simulink model "simulink_basic_blocks"  (R2022b)
settings: Solver=VariableStepAuto  StartTime=0.0  StopTime=10.0  RelTol=1e-3
settings Model: Creator=Soliman Rabie  LastModifiedBy=Soliman Rabie

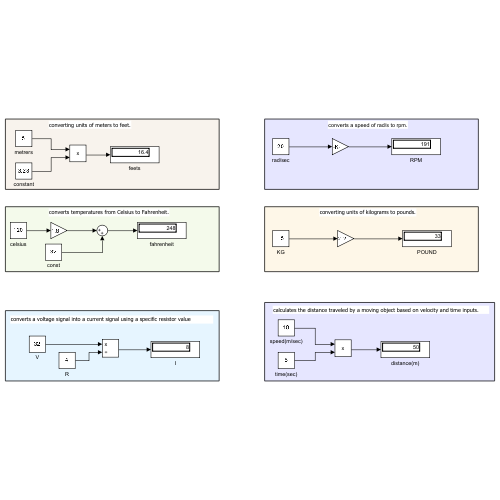
[thumbnail: Simulink's stored preview of the top-level diagram]
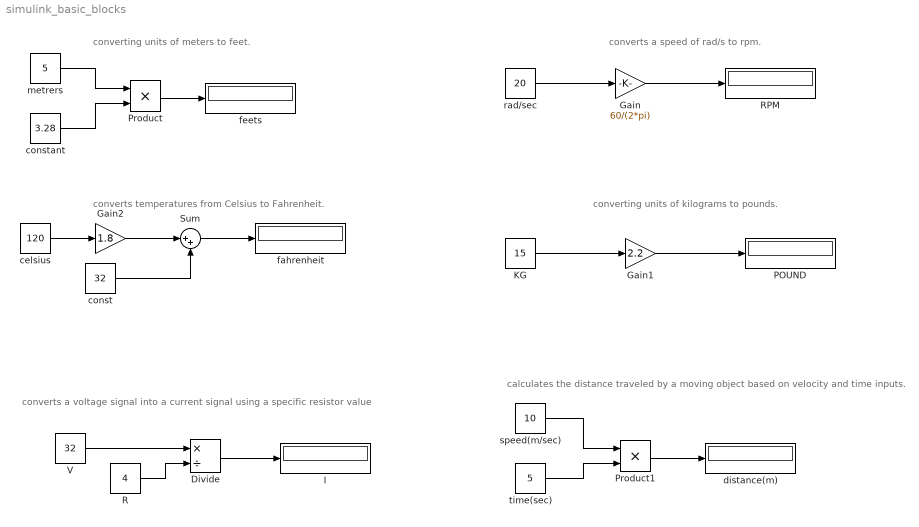
== system simulink_basic_blocks ==
  note: calculates the distance traveled by a moving object based on velocity and time inputs.
  note: converts a voltage signal into a current signal using a specific resistor value
  note: converting units of kilograms to pounds.
  note: converts temperatures from Celsius to Fahrenheit.
  note: converts a speed of rad/s to rpm.
  note: converting units of meters to feet.
  Divide : Product  Inputs=*/  RndMeth=Zero  SaturateOnIntegerOverflow=on
  Gain : Gain  Gain=60/(2*pi)
  Gain1 : Gain  Gain=2.2
  Gain2 : Gain  Gain=1.8
  I : Display
  KG : Constant  Value=15
  POUND : Display
  Product : Product
  Product1 : Product
  R : Constant  Value=4
  RPM : Display
  Sum : Sum  Inputs=|++
  V : Constant  Value=32
  celsius : Constant  Value=120
  const : Constant  Value=32
  constant : Constant  Value=3.28
  distance(m) : Display
  fahrenheit : Display
  feets : Display
  metrers : Constant  Value=5
  rad/sec : Constant  Value=20
  speed(m/sec) : Constant  Value=10
  time(sec) : Constant  Value=5
  wires:
  metrers/1 -> Product/1
  constant/1 -> Product/2
  Product/1 -> feets/1
  rad/sec/1 -> Gain/1
  Gain/1 -> RPM/1
  celsius/1 -> Gain2/1
  Gain2/1 -> Sum/1
  const/1 -> Sum/2
  Sum/1 -> fahrenheit/1
  Gain1/1 -> POUND/1
  KG/1 -> Gain1/1
  V/1 -> Divide/1
  Divide/1 -> I/1
  R/1 -> Divide/2
  time(sec)/1 -> Product1/2
  speed(m/sec)/1 -> Product1/1
  Product1/1 -> distance(m)/1
